simulink model "swps_3"  (Simulink 7.4)
settings: Solver=ode23s  StartTime=0.0  StopTime=.01  MaxStep=.1/50e3  RelTol=1e-3  AbsTol=1e-3
libraries: powerlib x15, simulink x4, simulink_extras x1
CloseFcn:
  | rtwprivate ssgencode ModelCloseRequest swps_2
settings Model: Creator=Owner  LastModifiedBy=Dick
settings SolverCC: InitialStep=1e-9
settings DataIOCC: LimitDataPoints=off  SaveOutput=off  SignalLogging=off  SaveTime=off  SignalLoggingName=sigsOut
settings OptimizationCC: BooleanDataType=off  InitFltsAndDblsToZero=on  OptimizeModelRefInitCode=on  LifeSpan=1
settings DebuggingCC: SaveWithParameterizedLinksMsg=none  SignalResolutionControl=TryResolveAllWithWarning  SolverPrmCheckMsg=none  MultiTaskDSMMsg=warning  MultiTaskCondExecSysMsg=none  StrictBusMsg=None
settings RTWCC: SystemTargetFile=ert.tlc  TemplateMakefile=ert_default_tmf  Description=Real-Time Workshop Embedded Coder (no auto configuration)  GenerateReport=on  ProcessScript=ert_make_rtw_hook  IncludeHyperlinkInReport=on  LaunchReport=on  IncludeERTFirstTime=on
settings CodeAppCC: IgnoreCustomStorageClasses=off
settings ERTTargetCC: TargetFcnLib=ansi_tfl_tmw.mat  MultiwordLength=2048  GenerateSampleERTMain=on  GenerateErtSFunction=on  InlinedParameterPlacement=NonHierarchical  ERTCustomFileTemplate=example_file_process.tlc  ConvertIfToSwitch=off

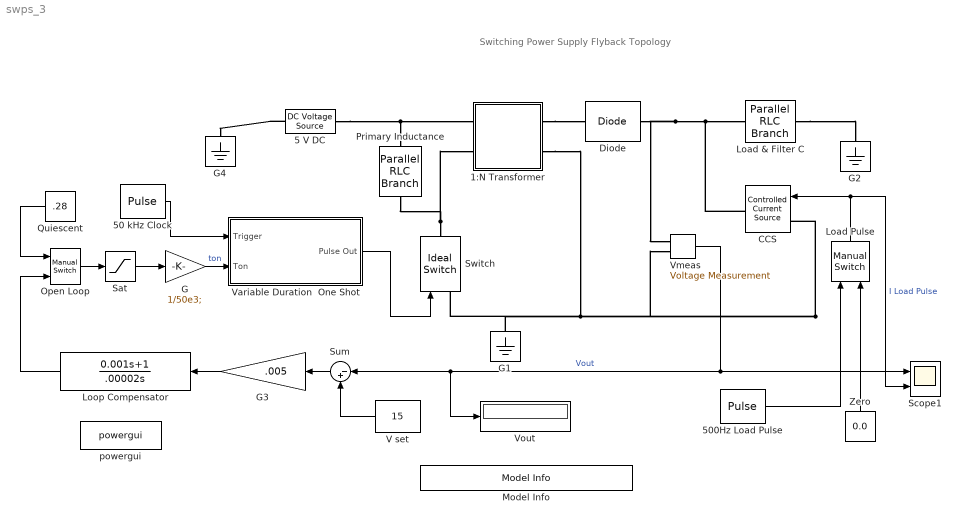
== system swps_3 ==
  note: Switching Power Supply
      | Flyback Topology
  1:N Transformer : Subsystem  mask{N=-3}
      mask prompts: N "Turns Ratio Secondary/Primary"
  5 V DC : powerlib/Electrical Sources/DC Voltage Source  Description=source block  DialogController=POWERSYS.PowerSysDialog  SystemSampleTime=-1  Amplitude=5  Measurements=None
      settings: AttributesFormatString=\n
  50 kHz Clock : DiscretePulseGenerator  PulseType=Time based  Amplitude=1  Period=1/50e3;  PulseWidth=50  PhaseDelay=1e-6  SampleTime=1
  500Hz Load Pulse : DiscretePulseGenerator  PulseType=Time based  Amplitude=-1  Period=1/500  PulseWidth=50  PhaseDelay=1e-6  SampleTime=1
  CCS : powerlib/Electrical Sources/Controlled Current Source  Description=source block  DialogController=POWERSYS.PowerSysDialog  SystemSampleTime=-1  Initialize=off  Source_Type=AC  Amplitude=10  Phase=0  Frequency=0  Measurements=None
      settings: AttributesFormatString=\n
  Diode : powerlib/Power Electronics/Diode  DialogController=POWERSYS.PowerSysDialog  SystemSampleTime=-1  Ron=1  Lon=0  Vf=.25  IC=0  UseSnubber=off  Rs=inf  Cs=0  Measurements=off
  G : Gain  Gain=1/50e3;  ParameterDataType=sfix(16)  ParameterScaling=2^0  OutDataType=sfix(16)  OutScaling=2^0  SaturateOnIntegerOverflow=on  OutDataTypeStr=Inherit: Same as input  ParamDataTypeStr=Inherit: Same as input
  G1 : powerlib/Elements/Ground  DialogController=POWERSYS.PowerSysDialog  PhysicalDomain=powersysdomain  SubClassName=unknown  LeftPortType=p1  RightPortType=p1  LConnTagsString=a
  G2 : powerlib/Elements/Ground  DialogController=POWERSYS.PowerSysDialog  PhysicalDomain=powersysdomain  SubClassName=unknown  LeftPortType=p1  RightPortType=p1  LConnTagsString=a
  G3 : Gain  Gain=.005  ParameterDataType=sfix(16)  ParameterScaling=2^0  OutDataType=sfix(16)  OutScaling=2^0  SaturateOnIntegerOverflow=on  OutDataTypeStr=Inherit: Same as input  ParamDataTypeStr=Inherit: Same as input
  G4 : powerlib/Elements/Ground  DialogController=POWERSYS.PowerSysDialog  PhysicalDomain=powersysdomain  SubClassName=unknown  LeftPortType=p1  RightPortType=p1  LConnTagsString=a
  Load & Filter C : powerlib/Elements/Parallel RLC Branch  DialogController=POWERSYS.PowerSysDialog  PhysicalDomain=powersysdomain  SubClassName=unknown  LeftPortType=p1  RightPortType=p1  LConnTagsString=a  RConnTagsString=__new0  BranchType=RC  Resistance=15  Inductance=1.0  SetiL0=off  InitialCurrent=0  Capacitance=100e-6  Setx0=off  InitialVoltage=0  Measurements=None
  Load Pulse : simulink/Signal Routing/Manual Switch  SystemSampleTime=-1  sw=1  action=0  varsize=off
  Loop Compensator : TransferFcn  Numerator=[ 0.001 1]  Denominator=[.00002 0]
  Model Info : simulink/Model-Wide Utilities/Model Info  SystemSampleTime=-1  InitialBlockCM=None  BlockCM=None  Frame=on  DisplayStringWithTags=Copywrite 2005-2010 The MathWorks, Inc.  HorizontalTextAlignment=Center  LeftAlignmentValue=0.5  SourceBlockDiagram=swps_3  TagMaxNumber=20
  Open Loop : simulink/Signal Routing/Manual Switch  SystemSampleTime=-1  sw=0  action=0  varsize=off
  Primary Inductance : powerlib/Elements/Parallel RLC Branch  DialogController=POWERSYS.PowerSysDialog  PhysicalDomain=powersysdomain  SubClassName=unknown  LeftPortType=p1  RightPortType=p1  LConnTagsString=a  RConnTagsString=__new0  BranchType=RL  Resistance=1000  Inductance=1e-6  SetiL0=off  InitialCurrent=0  Capacitance=1.0  Setx0=off  InitialVoltage=0  Measurements=None
  Quiescent : Constant  Value=.28  OutDataType=sfix(16)  OutScaling=2^0
  Sat : Saturate  UpperLimit=0.65  LowerLimit=.01
  Scope1 : Scope  NumInputPorts=2
      settings: TimeRange=0.01  YMin=0~-2  YMax=22.5~1  SaveName=ScopeData2
  Sum : Sum  Inputs=|-+  OutDataType=sfix(16)  OutScaling=2^0  SaturateOnIntegerOverflow=on  InputSameDT=on  OutDataTypeStr=Inherit: Same as first input
  Switch : powerlib/Power Electronics/Ideal Switch  DialogController=POWERSYS.PowerSysDialog  SystemSampleTime=-1  Ron=0.01  Lon=0  IC=0  Rs=0  Cs=0  Measurements=off
      settings: AttributesFormatString=\n
  "V set " : Constant  Value=15  OutDataType=sfix(16)  OutScaling=2^0
  Variable Duration  One Shot : Subsystem
  Vmeas : powerlib/Measurements/Voltage Measurement  Tag=PoWeRsYsTeMmEaSuReMeNt  DialogController=POWERSYS.PowerSysDialog  SystemSampleTime=-1  PhasorSimulation=off  OutputType=Magnitude  PSBequivalent=0
  Vout : Display
      settings: Decimation=20
  Zero : Constant  Value=0.0  OutDataType=sfix(16)  OutScaling=2^0
  powergui : powerlib/powergui  SystemSampleTime=-1  SimulationMode=Continuous  SampleTime=0  frequency=60  SPID=off  DisableSnubberDevices=off  DisableRonSwitches=off  DisableVfSwitches=off  SwTol=0  Interpol=off  frequencyindice=0  echomessages=off  HookPort=off  DisplayEquations=off  FunctionMessages=off  EnableUseOfTLC=off  x0status=blocks  RestoreLinks=warning  Frange=[0:2:500]  Ylog=off  Xlog=on  ShowGrid=off  save=off  variable=ZData  ZoomFFT=on  StartTime=0.0  cycles=1  DisplayStyle=1  fundamental=60  FreqAxis=off  MaxFrequency=1000  frequencyindicesteady=1  RmsSteady=1  display=off  Ts=0  methode=off
  wires:
  50 kHz Clock/1 -> Variable Duration  One Shot/1(Trigger)
  Sum/1 -> G3/1
  "V set "/1 -> Sum/2
  Quiescent/1 -> Open Loop/1
  Open Loop/1 -> Sat/1
  G/1 -> Variable Duration  One Shot/2(Ton)  "ton"
  500Hz Load Pulse/1 -> Load Pulse/1
  Zero/1 -> Load Pulse/2
  G3/1 -> Loop Compensator/1
  Vmeas/1 -> Scope1/1, Sum/1, Vout/1  "Vout"
  Load Pulse/1 -> CCS/1, Scope1/2  "I Load Pulse"
  Loop Compensator/1 -> Open Loop/2
  Variable Duration  One Shot/1(Pulse Out) -> Switch/1
  Sat/1 -> G/1
  connections:
  Load & Filter C/RConn1 -- G2/LConn1
  5 V DC/LConn1 -- G4/LConn1
  Primary Inductance/RConn1 -- Switch/RConn1 -- 1:N Transformer/LConn2
  Vmeas/LConn1 -- Diode/RConn1 -- Load & Filter C/LConn1 -- CCS/RConn1
  Switch/LConn1 -- 1:N Transformer/RConn2 -- G1/LConn1 -- CCS/LConn1 -- Vmeas/LConn2
  5 V DC/RConn1 -- Primary Inductance/LConn1 -- 1:N Transformer/LConn1
  1:N Transformer/RConn1 -- Diode/LConn1

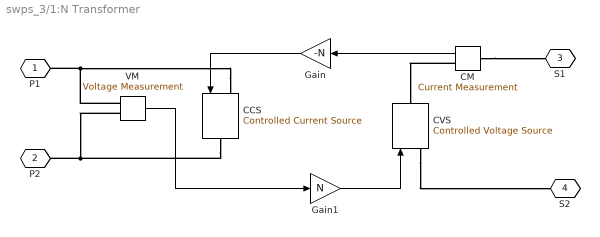
== system swps_3/1:N Transformer ==
  CCS : powerlib/Electrical Sources/Controlled Current Source  Description=source block  DialogController=POWERSYS.PowerSysDialog  SystemSampleTime=-1  Initialize=off  Source_Type=AC  Amplitude=0  Phase=0  Frequency=0  Measurements=None
      settings: AttributesFormatString=\n
  CM : powerlib/Measurements/Current Measurement  Tag=PoWeRsYsTeMmEaSuReMeNt  DialogController=POWERSYS.PowerSysDialog  SystemSampleTime=-1  PhasorSimulation=off  OutputType=Magnitude  PSBequivalent=0
  CVS : powerlib/Electrical Sources/Controlled Voltage Source  Description=source block  DialogController=POWERSYS.PowerSysDialog  SystemSampleTime=-1  Initialize=off  Source_Type=AC  Amplitude=0  Phase=0  Frequency=0  Measurements=None
      settings: AttributesFormatString=\n
  Gain : Gain  Gain=-N  ParameterDataType=sfix(16)  ParameterScaling=2^0  OutDataType=sfix(16)  OutScaling=2^0  SaturateOnIntegerOverflow=on  OutDataTypeStr=Inherit: Same as input  ParamDataTypeStr=Inherit: Same as input
  Gain1 : Gain  Gain=N  ParameterDataType=sfix(16)  ParameterScaling=2^0  OutDataType=sfix(16)  OutScaling=2^0  SaturateOnIntegerOverflow=on  OutDataTypeStr=Inherit: Same as input  ParamDataTypeStr=Inherit: Same as input
  VM : powerlib/Measurements/Voltage Measurement  Tag=PoWeRsYsTeMmEaSuReMeNt  DialogController=POWERSYS.PowerSysDialog  SystemSampleTime=-1  PhasorSimulation=off  OutputType=Magnitude  PSBequivalent=0
  P1 : PMIOPort  Tag=PMCPort  Port=1  Side=Left
  P2 : PMIOPort  Tag=PMCPort  Port=2  Side=Left
  S1 : PMIOPort  Tag=PMCPort  Port=3  Side=Right
  S2 : PMIOPort  Tag=PMCPort  Port=4  Side=Right
  wires:
  VM/1 -> Gain1/1
  Gain1/1 -> CVS/1
  Gain/1 -> CCS/1
  CM/1 -> Gain/1
  connections:
  CCS/LConn1 -- P1/RConn1 -- VM/LConn1
  CCS/RConn1 -- P2/RConn1 -- VM/LConn2
  CM/LConn1 -- S1/RConn1
  CM/RConn1 -- CVS/RConn1
  CVS/LConn1 -- S2/RConn1

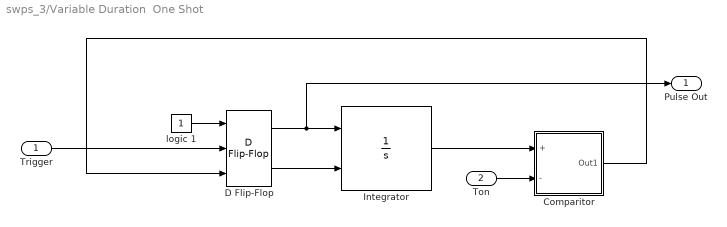
== system swps_3/Variable Duration  One Shot ==
  Trigger : Inport  OutDataType=sfix(16)  OutScaling=2^0
  Ton : Inport  Port=2  OutDataType=sfix(16)  OutScaling=2^0
  Comparitor : Subsystem
  D Flip-Flop : simulink_extras/Flip Flops/D Flip-Flop  SystemSampleTime=-1
  Integrator : Integrator  ExternalReset=level
  logic 1 : Constant  OutDataType=sfix(16)  OutScaling=2^0
  Pulse Out : Outport  OutDataType=sfix(16)  OutScaling=2^0
  wires:
  D Flip-Flop/2 -> Integrator/2
  logic 1/1 -> D Flip-Flop/1
  Integrator/1 -> Comparitor/1(+)
  D Flip-Flop/1 -> Integrator/1, Pulse Out/1
  Trigger/1 -> D Flip-Flop/2
  Ton/1 -> Comparitor/2(-)
  Comparitor/1(Out1) -> D Flip-Flop/3

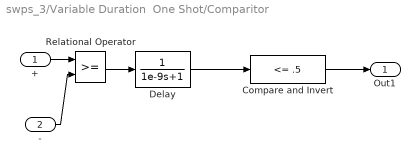
== system swps_3/Variable Duration  One Shot/Comparitor ==
  + : Inport  OutDataType=sfix(16)  OutScaling=2^0
  - : Inport  Port=2  OutDataType=sfix(16)  OutScaling=2^0
  "Compare and Invert " : simulink/Logic and Bit Operations/Compare To Constant  SystemSampleTime=-1  relop=<=  const=.5  LogicOutDataTypeMode=uint8  ZeroCross=off
  Delay : TransferFcn  Denominator=[1e-9 1]
  Relational Operator : RelationalOperator  InputSameDT=on
  Out1 : Outport  OutDataType=sfix(16)  OutScaling=2^0
  wires:
  Relational Operator/1 -> Delay/1
  +/1 -> Relational Operator/1
  Delay/1 -> "Compare and Invert "/1
  -/1 -> Relational Operator/2
  "Compare and Invert "/1 -> Out1/1
